simulink library "Filtlib"  (Simulink 7.7)
settings: Solver=ode45  StartTime=0.0  StopTime=10.0  RelTol=1e-3
settings Model: Creator=jzqwf2  LastModifiedBy=jzqwf2

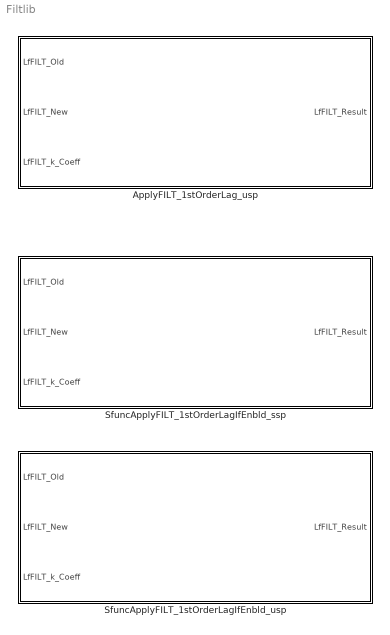
== system Filtlib ==
  ApplyFILT_1stOrderLag_usp : Subsystem  TreatAsAtomicUnit=on
      settings: RTWSystemCode=Inline
  SfuncApplyFILT_1stOrderLagIfEnbld_ssp : Subsystem  TreatAsAtomicUnit=on
      settings: RTWSystemCode=Inline
  SfuncApplyFILT_1stOrderLagIfEnbld_usp : Subsystem  TreatAsAtomicUnit=on
      settings: RTWSystemCode=Inline

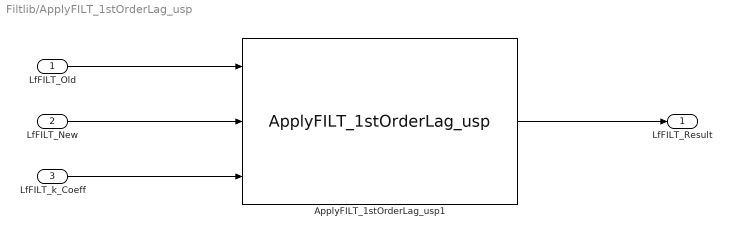
== system Filtlib/ApplyFILT_1stOrderLag_usp ==
  LfFILT_Old : Inport
  LfFILT_New : Inport  Port=2
  LfFILT_k_Coeff : Inport  Port=3
  ApplyFILT_1stOrderLag_usp1 : S-Function  FunctionName=ApplyFILT_1stOrderLag_usp  EnableBusSupport=off
  LfFILT_Result : Outport
  wires:
  LfFILT_Old/1 -> ApplyFILT_1stOrderLag_usp1/1
  ApplyFILT_1stOrderLag_usp1/1 -> LfFILT_Result/1
  LfFILT_k_Coeff/1 -> ApplyFILT_1stOrderLag_usp1/3
  LfFILT_New/1 -> ApplyFILT_1stOrderLag_usp1/2

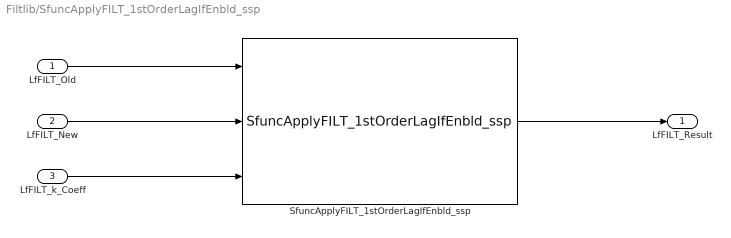
== system Filtlib/SfuncApplyFILT_1stOrderLagIfEnbld_ssp ==
  LfFILT_Old : Inport
  LfFILT_New : Inport  Port=2
  LfFILT_k_Coeff : Inport  Port=3
  SfuncApplyFILT_1stOrderLagIfEnbld_ssp : S-Function  FunctionName=SfuncApplyFILT_1stOrderLagIfEnbld_ssp  EnableBusSupport=off
  LfFILT_Result : Outport
  wires:
  LfFILT_New/1 -> SfuncApplyFILT_1stOrderLagIfEnbld_ssp/2
  LfFILT_k_Coeff/1 -> SfuncApplyFILT_1stOrderLagIfEnbld_ssp/3
  SfuncApplyFILT_1stOrderLagIfEnbld_ssp/1 -> LfFILT_Result/1
  LfFILT_Old/1 -> SfuncApplyFILT_1stOrderLagIfEnbld_ssp/1

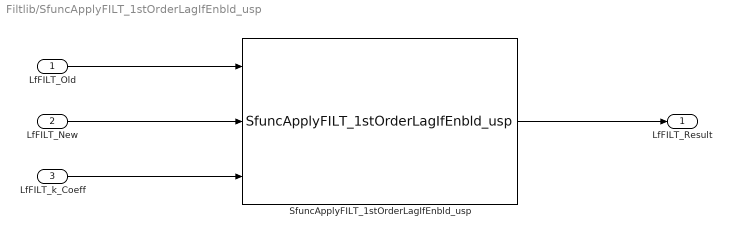
== system Filtlib/SfuncApplyFILT_1stOrderLagIfEnbld_usp ==
  LfFILT_Old : Inport
  LfFILT_New : Inport  Port=2
  LfFILT_k_Coeff : Inport  Port=3
  SfuncApplyFILT_1stOrderLagIfEnbld_usp : S-Function  FunctionName=SfuncApplyFILT_1stOrderLagIfEnbld_usp  EnableBusSupport=off
  LfFILT_Result : Outport
  wires:
  SfuncApplyFILT_1stOrderLagIfEnbld_usp/1 -> LfFILT_Result/1
  LfFILT_Old/1 -> SfuncApplyFILT_1stOrderLagIfEnbld_usp/1
  LfFILT_New/1 -> SfuncApplyFILT_1stOrderLagIfEnbld_usp/2
  LfFILT_k_Coeff/1 -> SfuncApplyFILT_1stOrderLagIfEnbld_usp/3
